simulink model "final_test1"  (Simulink 7.7)
settings: Solver=ode45  StartTime=0.0  StopTime=10.0  RelTol=1e-3
undefined symbols (not defined in the file): des_attributefunction_support, des_figposition
libraries: simeventsattributes2 x107, simeventsserver1 x73, simeventstranslate1 x43, simeventsrouting1 x28, commrandsrc2 x18, simeventsgenerators1 x12, simeventssink1 x9, simeventsqueue1 x6, simulink_extras x1, simeventssignalmanage1 x1
(part 3 of 5)

== system final_test1/Red Link2 ==
  Attribute Function : Subsystem  LoadFcn=des_attributefunction_support(gcb,'LoadFcn');  StartFcn=des_attributefunction_support(gcb,'StartFcn');  mask(Attribute Function){OutputNamePrefix=out_}
      mask prompts: OutputNamePrefix "Prefix name"
      settings: CopyFcn=des_attributefunction_support(gcb,'CopyFcn');  OpenFcn=des_attributefunction_support(gcb,'OpenFcn');  ErrorFcn=des_error_redirect
      mask Help: helpview(simeventsbhelp('attributefunction'))
      mask Display: image(des_iconLoad('attribFunction.jpg'),'center');
  Attribute Function1 : Subsystem  LoadFcn=des_attributefunction_support(gcb,'LoadFcn');  StartFcn=des_attributefunction_support(gcb,'StartFcn');  mask(Attribute Function){OutputNamePrefix=out_}
      mask prompts: OutputNamePrefix "Prefix name"
      settings: CopyFcn=des_attributefunction_support(gcb,'CopyFcn');  OpenFcn=des_attributefunction_support(gcb,'OpenFcn');  ErrorFcn=des_error_redirect
      mask Help: helpview(simeventsbhelp('attributefunction'))
      mask Display: image(des_iconLoad('attribFunction.jpg'),'center');
  Infinite Server : simeventsserver1/Infinite Server  SystemSampleTime=-1  ServiceTimeFrom=Dialog  ServiceTime=0.001  AttributeName=ServiceTime  PriorityServiceCompletion=500  EnableTOPort=off  StatNumberDeparted=Off  StatNumberInBlock=Off  StatPendingEntity=Off  StatNumberPending=Off  StatAverageWait=Off  StatNumberTimedout=Off
  Infinite Server1 : simeventsserver1/Infinite Server  SystemSampleTime=-1  ServiceTimeFrom=Dialog  ServiceTime=0.001  AttributeName=ServiceTime  PriorityServiceCompletion=500  EnableTOPort=off  StatNumberDeparted=Off  StatNumberInBlock=Off  StatPendingEntity=Off  StatNumberPending=Off  StatAverageWait=Off  StatNumberTimedout=Off
  Single Server : simeventsserver1/Single Server  SystemSampleTime=-1  ServiceTimeFrom=Attribute  ServiceTime=1  AttributeName=ServiceTime  PriorityServiceCompletion=500  PermitPreemption=off  SortingAttributeName=PriorityAttributeName  SortingDirection=Ascending  WriteToAttribute=off  ResidualAttributeName=ResidualServiceTime  CreateAttribute=on  EnableTOPort=off  StatNumberDeparted=Off  StatNumberInBlock=Off  StatNumberPreempted=Off  StatPendingEntity=Off  StatAverageWait=Off  StatUtilization=Off  StatNumberTimedout=Off
  Single Server1 : simeventsserver1/Single Server  SystemSampleTime=-1  ServiceTimeFrom=Attribute  ServiceTime=1  AttributeName=ServiceTime  PriorityServiceCompletion=500  PermitPreemption=off  SortingAttributeName=PriorityAttributeName  SortingDirection=Ascending  WriteToAttribute=off  ResidualAttributeName=ResidualServiceTime  CreateAttribute=on  EnableTOPort=off  StatNumberDeparted=Off  StatNumberInBlock=Off  StatNumberPreempted=Off  StatPendingEntity=Off  StatAverageWait=Off  StatUtilization=Off  StatNumberTimedout=Off
  Input1 : PMIOPort  Port=1  Side=Left
  Output1 : PMIOPort  Port=2  Side=Right
  Input2 : PMIOPort  Port=3  Side=Right
  Output2 : PMIOPort  Port=4  Side=Left
  connections:
  Input1/RConn1 -- Attribute Function/LConn1
  Output1/RConn1 -- Infinite Server1/RConn1
  Output2/RConn1 -- Infinite Server/RConn1
  Attribute Function/RConn1 -- Single Server/LConn1
  Single Server/RConn1 -- Infinite Server1/LConn1
  Single Server1/RConn1 -- Infinite Server/LConn1
  Input2/RConn1 -- Attribute Function1/LConn1
  Attribute Function1/RConn1 -- Single Server1/LConn1

== system final_test1/Red Link3 ==
  Attribute Function : Subsystem  LoadFcn=des_attributefunction_support(gcb,'LoadFcn');  StartFcn=des_attributefunction_support(gcb,'StartFcn');  mask(Attribute Function){OutputNamePrefix=out_}
      mask prompts: OutputNamePrefix "Prefix name"
      settings: CopyFcn=des_attributefunction_support(gcb,'CopyFcn');  OpenFcn=des_attributefunction_support(gcb,'OpenFcn');  ErrorFcn=des_error_redirect
      mask Help: helpview(simeventsbhelp('attributefunction'))
      mask Display: image(des_iconLoad('attribFunction.jpg'),'center');
  Attribute Function1 : Subsystem  LoadFcn=des_attributefunction_support(gcb,'LoadFcn');  StartFcn=des_attributefunction_support(gcb,'StartFcn');  mask(Attribute Function){OutputNamePrefix=out_}
      mask prompts: OutputNamePrefix "Prefix name"
      settings: CopyFcn=des_attributefunction_support(gcb,'CopyFcn');  OpenFcn=des_attributefunction_support(gcb,'OpenFcn');  ErrorFcn=des_error_redirect
      mask Help: helpview(simeventsbhelp('attributefunction'))
      mask Display: image(des_iconLoad('attribFunction.jpg'),'center');
  Infinite Server : simeventsserver1/Infinite Server  SystemSampleTime=-1  ServiceTimeFrom=Dialog  ServiceTime=0.001  AttributeName=ServiceTime  PriorityServiceCompletion=500  EnableTOPort=off  StatNumberDeparted=Off  StatNumberInBlock=Off  StatPendingEntity=Off  StatNumberPending=Off  StatAverageWait=Off  StatNumberTimedout=Off
  Infinite Server1 : simeventsserver1/Infinite Server  SystemSampleTime=-1  ServiceTimeFrom=Dialog  ServiceTime=0.001  AttributeName=ServiceTime  PriorityServiceCompletion=500  EnableTOPort=off  StatNumberDeparted=Off  StatNumberInBlock=Off  StatPendingEntity=Off  StatNumberPending=Off  StatAverageWait=Off  StatNumberTimedout=Off
  Single Server : simeventsserver1/Single Server  SystemSampleTime=-1  ServiceTimeFrom=Attribute  ServiceTime=1  AttributeName=ServiceTime  PriorityServiceCompletion=500  PermitPreemption=off  SortingAttributeName=PriorityAttributeName  SortingDirection=Ascending  WriteToAttribute=off  ResidualAttributeName=ResidualServiceTime  CreateAttribute=on  EnableTOPort=off  StatNumberDeparted=Off  StatNumberInBlock=Off  StatNumberPreempted=Off  StatPendingEntity=Off  StatAverageWait=Off  StatUtilization=Off  StatNumberTimedout=Off
  Single Server1 : simeventsserver1/Single Server  SystemSampleTime=-1  ServiceTimeFrom=Attribute  ServiceTime=1  AttributeName=ServiceTime  PriorityServiceCompletion=500  PermitPreemption=off  SortingAttributeName=PriorityAttributeName  SortingDirection=Ascending  WriteToAttribute=off  ResidualAttributeName=ResidualServiceTime  CreateAttribute=on  EnableTOPort=off  StatNumberDeparted=Off  StatNumberInBlock=Off  StatNumberPreempted=Off  StatPendingEntity=Off  StatAverageWait=Off  StatUtilization=Off  StatNumberTimedout=Off
  Input1 : PMIOPort  Port=1  Side=Left
  Output1 : PMIOPort  Port=2  Side=Right
  Input2 : PMIOPort  Port=3  Side=Right
  Output2 : PMIOPort  Port=4  Side=Left
  connections:
  Attribute Function1/RConn1 -- Single Server1/LConn1
  Input2/RConn1 -- Attribute Function1/LConn1
  Single Server1/RConn1 -- Infinite Server/LConn1
  Single Server/RConn1 -- Infinite Server1/LConn1
  Attribute Function/RConn1 -- Single Server/LConn1
  Output2/RConn1 -- Infinite Server/RConn1
  Output1/RConn1 -- Infinite Server1/RConn1
  Input1/RConn1 -- Attribute Function/LConn1

== system final_test1/Red Link4 ==
  Attribute Function : Subsystem  LoadFcn=des_attributefunction_support(gcb,'LoadFcn');  StartFcn=des_attributefunction_support(gcb,'StartFcn');  mask(Attribute Function){OutputNamePrefix=out_}
      mask prompts: OutputNamePrefix "Prefix name"
      settings: CopyFcn=des_attributefunction_support(gcb,'CopyFcn');  OpenFcn=des_attributefunction_support(gcb,'OpenFcn');  ErrorFcn=des_error_redirect
      mask Help: helpview(simeventsbhelp('attributefunction'))
      mask Display: image(des_iconLoad('attribFunction.jpg'),'center');
  Attribute Function1 : Subsystem  LoadFcn=des_attributefunction_support(gcb,'LoadFcn');  StartFcn=des_attributefunction_support(gcb,'StartFcn');  mask(Attribute Function){OutputNamePrefix=out_}
      mask prompts: OutputNamePrefix "Prefix name"
      settings: CopyFcn=des_attributefunction_support(gcb,'CopyFcn');  OpenFcn=des_attributefunction_support(gcb,'OpenFcn');  ErrorFcn=des_error_redirect
      mask Help: helpview(simeventsbhelp('attributefunction'))
      mask Display: image(des_iconLoad('attribFunction.jpg'),'center');
  Infinite Server : simeventsserver1/Infinite Server  SystemSampleTime=-1  ServiceTimeFrom=Dialog  ServiceTime=0.001  AttributeName=ServiceTime  PriorityServiceCompletion=500  EnableTOPort=off  StatNumberDeparted=Off  StatNumberInBlock=Off  StatPendingEntity=Off  StatNumberPending=Off  StatAverageWait=Off  StatNumberTimedout=Off
  Infinite Server1 : simeventsserver1/Infinite Server  SystemSampleTime=-1  ServiceTimeFrom=Dialog  ServiceTime=0.001  AttributeName=ServiceTime  PriorityServiceCompletion=500  EnableTOPort=off  StatNumberDeparted=Off  StatNumberInBlock=Off  StatPendingEntity=Off  StatNumberPending=Off  StatAverageWait=Off  StatNumberTimedout=Off
  Single Server : simeventsserver1/Single Server  SystemSampleTime=-1  ServiceTimeFrom=Attribute  ServiceTime=1  AttributeName=ServiceTime  PriorityServiceCompletion=500  PermitPreemption=off  SortingAttributeName=PriorityAttributeName  SortingDirection=Ascending  WriteToAttribute=off  ResidualAttributeName=ResidualServiceTime  CreateAttribute=on  EnableTOPort=off  StatNumberDeparted=Off  StatNumberInBlock=Off  StatNumberPreempted=Off  StatPendingEntity=Off  StatAverageWait=Off  StatUtilization=Off  StatNumberTimedout=Off
  Single Server1 : simeventsserver1/Single Server  SystemSampleTime=-1  ServiceTimeFrom=Attribute  ServiceTime=1  AttributeName=ServiceTime  PriorityServiceCompletion=500  PermitPreemption=off  SortingAttributeName=PriorityAttributeName  SortingDirection=Ascending  WriteToAttribute=off  ResidualAttributeName=ResidualServiceTime  CreateAttribute=on  EnableTOPort=off  StatNumberDeparted=Off  StatNumberInBlock=Off  StatNumberPreempted=Off  StatPendingEntity=Off  StatAverageWait=Off  StatUtilization=Off  StatNumberTimedout=Off
  Input1 : PMIOPort  Port=1  Side=Left
  Output1 : PMIOPort  Port=2  Side=Right
  Input2 : PMIOPort  Port=3  Side=Right
  Output2 : PMIOPort  Port=4  Side=Left
  connections:
  Input1/RConn1 -- Attribute Function/LConn1
  Output1/RConn1 -- Infinite Server1/RConn1
  Output2/RConn1 -- Infinite Server/RConn1
  Attribute Function/RConn1 -- Single Server/LConn1
  Single Server/RConn1 -- Infinite Server1/LConn1
  Single Server1/RConn1 -- Infinite Server/LConn1
  Input2/RConn1 -- Attribute Function1/LConn1
  Attribute Function1/RConn1 -- Single Server1/LConn1

== system final_test1/Red Link5 ==
  Attribute Function : Subsystem  LoadFcn=des_attributefunction_support(gcb,'LoadFcn');  StartFcn=des_attributefunction_support(gcb,'StartFcn');  mask(Attribute Function){OutputNamePrefix=out_}
      mask prompts: OutputNamePrefix "Prefix name"
      settings: CopyFcn=des_attributefunction_support(gcb,'CopyFcn');  OpenFcn=des_attributefunction_support(gcb,'OpenFcn');  ErrorFcn=des_error_redirect
      mask Help: helpview(simeventsbhelp('attributefunction'))
      mask Display: image(des_iconLoad('attribFunction.jpg'),'center');
  Attribute Function1 : Subsystem  LoadFcn=des_attributefunction_support(gcb,'LoadFcn');  StartFcn=des_attributefunction_support(gcb,'StartFcn');  mask(Attribute Function){OutputNamePrefix=out_}
      mask prompts: OutputNamePrefix "Prefix name"
      settings: CopyFcn=des_attributefunction_support(gcb,'CopyFcn');  OpenFcn=des_attributefunction_support(gcb,'OpenFcn');  ErrorFcn=des_error_redirect
      mask Help: helpview(simeventsbhelp('attributefunction'))
      mask Display: image(des_iconLoad('attribFunction.jpg'),'center');
  Infinite Server : simeventsserver1/Infinite Server  SystemSampleTime=-1  ServiceTimeFrom=Dialog  ServiceTime=0.001  AttributeName=ServiceTime  PriorityServiceCompletion=500  EnableTOPort=off  StatNumberDeparted=Off  StatNumberInBlock=Off  StatPendingEntity=Off  StatNumberPending=Off  StatAverageWait=Off  StatNumberTimedout=Off
  Infinite Server1 : simeventsserver1/Infinite Server  SystemSampleTime=-1  ServiceTimeFrom=Dialog  ServiceTime=0.001  AttributeName=ServiceTime  PriorityServiceCompletion=500  EnableTOPort=off  StatNumberDeparted=Off  StatNumberInBlock=Off  StatPendingEntity=Off  StatNumberPending=Off  StatAverageWait=Off  StatNumberTimedout=Off
  Single Server : simeventsserver1/Single Server  SystemSampleTime=-1  ServiceTimeFrom=Attribute  ServiceTime=1  AttributeName=ServiceTime  PriorityServiceCompletion=500  PermitPreemption=off  SortingAttributeName=PriorityAttributeName  SortingDirection=Ascending  WriteToAttribute=off  ResidualAttributeName=ResidualServiceTime  CreateAttribute=on  EnableTOPort=off  StatNumberDeparted=Off  StatNumberInBlock=Off  StatNumberPreempted=Off  StatPendingEntity=Off  StatAverageWait=Off  StatUtilization=Off  StatNumberTimedout=Off
  Single Server1 : simeventsserver1/Single Server  SystemSampleTime=-1  ServiceTimeFrom=Attribute  ServiceTime=1  AttributeName=ServiceTime  PriorityServiceCompletion=500  PermitPreemption=off  SortingAttributeName=PriorityAttributeName  SortingDirection=Ascending  WriteToAttribute=off  ResidualAttributeName=ResidualServiceTime  CreateAttribute=on  EnableTOPort=off  StatNumberDeparted=Off  StatNumberInBlock=Off  StatNumberPreempted=Off  StatPendingEntity=Off  StatAverageWait=Off  StatUtilization=Off  StatNumberTimedout=Off
  Input1 : PMIOPort  Port=1  Side=Left
  Output1 : PMIOPort  Port=2  Side=Right
  Input2 : PMIOPort  Port=3  Side=Right
  Output2 : PMIOPort  Port=4  Side=Left
  connections:
  Attribute Function1/RConn1 -- Single Server1/LConn1
  Input2/RConn1 -- Attribute Function1/LConn1
  Single Server1/RConn1 -- Infinite Server/LConn1
  Single Server/RConn1 -- Infinite Server1/LConn1
  Attribute Function/RConn1 -- Single Server/LConn1
  Output2/RConn1 -- Infinite Server/RConn1
  Output1/RConn1 -- Infinite Server1/RConn1
  Input1/RConn1 -- Attribute Function/LConn1

== system final_test1/Blue Link/Attribute Function ==
  Embedded MATLAB Function : Stateflow chart  TreatAsAtomicUnit=on
      settings: PropExecContextOutsideSubsystem=on
  __DEML__EDE2FCE__ : simeventstranslate1/Entity Departure Event to Function-Call Event  Priority=1  SystemSampleTime=-1  TimingFunctionCallF1=Before entity departure  EnableE1Port=off  EnableF2Port=off  TimingFunctionCallF2=Before entity departure  EnableE2Port=off  StatNumberDeparted=Off  StatNumberF1Calls=Off  StatNumberF2Calls=Off  IsInsideAFB=on
  __DEML__GA__ : simeventsattributes2/Get Attribute  Priority=1  SystemSampleTime=-1  AttributeName=length  AttributeMissing=Error  AttributeDefaultValue=1  AttributeSendTiming=Before entity departure  AttributeTreatAsVector=1  StatNumberDeparted=Off  EvaluatedDefaultAttributeValue={[]}
  __DEML__SA__ : simeventsattributes2/Set Attribute  Priority=1  SystemSampleTime=-1  AttributeFrom=Signal port  AttributeName=ServiceTime  AttributeTreatAsVector=1  AttributeValue=1  AttributeCreate=on  StatNumberDeparted=Off  EvaluatedAttributeValue={[]}
  IN : PMIOPort  Port=1  Side=Left
  OUT : PMIOPort  Port=2  Side=Right
  wires:
  __DEML__EDE2FCE__/1 -> Embedded MATLAB Function/Trigger
  __DEML__GA__/1 -> Embedded MATLAB Function/1(length)
  Embedded MATLAB Function/1(out_ServiceTime) -> __DEML__SA__/1
  connections:
  __DEML__EDE2FCE__/RConn1 -- __DEML__SA__/LConn1
  __DEML__GA__/RConn1 -- __DEML__EDE2FCE__/LConn1
  IN/RConn1 -- __DEML__GA__/LConn1
  __DEML__SA__/RConn1 -- OUT/RConn1

== system final_test1/Blue Link/Attribute Function1 ==
  Embedded MATLAB Function : Stateflow chart  TreatAsAtomicUnit=on
      settings: PropExecContextOutsideSubsystem=on
  __DEML__EDE2FCE__ : simeventstranslate1/Entity Departure Event to Function-Call Event  Priority=1  SystemSampleTime=-1  TimingFunctionCallF1=Before entity departure  EnableE1Port=off  EnableF2Port=off  TimingFunctionCallF2=Before entity departure  EnableE2Port=off  StatNumberDeparted=Off  StatNumberF1Calls=Off  StatNumberF2Calls=Off  IsInsideAFB=on
  __DEML__GA__ : simeventsattributes2/Get Attribute  Priority=1  SystemSampleTime=-1  AttributeName=length  AttributeMissing=Error  AttributeDefaultValue=1  AttributeSendTiming=Before entity departure  AttributeTreatAsVector=1  StatNumberDeparted=Off  EvaluatedDefaultAttributeValue={[]}
  __DEML__SA__ : simeventsattributes2/Set Attribute  Priority=1  SystemSampleTime=-1  AttributeFrom=Signal port  AttributeName=ServiceTime  AttributeTreatAsVector=1  AttributeValue=1  AttributeCreate=on  StatNumberDeparted=Off  EvaluatedAttributeValue={[]}
  IN : PMIOPort  Port=1  Side=Left
  OUT : PMIOPort  Port=2  Side=Right
  wires:
  __DEML__EDE2FCE__/1 -> Embedded MATLAB Function/Trigger
  __DEML__GA__/1 -> Embedded MATLAB Function/1(length)
  Embedded MATLAB Function/1(out_ServiceTime) -> __DEML__SA__/1
  connections:
  __DEML__SA__/RConn1 -- OUT/RConn1
  IN/RConn1 -- __DEML__GA__/LConn1
  __DEML__GA__/RConn1 -- __DEML__EDE2FCE__/LConn1
  __DEML__EDE2FCE__/RConn1 -- __DEML__SA__/LConn1

== system final_test1/Blue Link1/Attribute Function ==
  Embedded MATLAB Function : Stateflow chart  TreatAsAtomicUnit=on
      settings: PropExecContextOutsideSubsystem=on
  __DEML__EDE2FCE__ : simeventstranslate1/Entity Departure Event to Function-Call Event  Priority=1  SystemSampleTime=-1  TimingFunctionCallF1=Before entity departure  EnableE1Port=off  EnableF2Port=off  TimingFunctionCallF2=Before entity departure  EnableE2Port=off  StatNumberDeparted=Off  StatNumberF1Calls=Off  StatNumberF2Calls=Off  IsInsideAFB=on
  __DEML__GA__ : simeventsattributes2/Get Attribute  Priority=1  SystemSampleTime=-1  AttributeName=length  AttributeMissing=Error  AttributeDefaultValue=1  AttributeSendTiming=Before entity departure  AttributeTreatAsVector=1  StatNumberDeparted=Off  EvaluatedDefaultAttributeValue={[]}
  __DEML__SA__ : simeventsattributes2/Set Attribute  Priority=1  SystemSampleTime=-1  AttributeFrom=Signal port  AttributeName=ServiceTime  AttributeTreatAsVector=1  AttributeValue=1  AttributeCreate=on  StatNumberDeparted=Off  EvaluatedAttributeValue={[]}
  IN : PMIOPort  Port=1  Side=Left
  OUT : PMIOPort  Port=2  Side=Right
  wires:
  __DEML__EDE2FCE__/1 -> Embedded MATLAB Function/Trigger
  __DEML__GA__/1 -> Embedded MATLAB Function/1(length)
  Embedded MATLAB Function/1(out_ServiceTime) -> __DEML__SA__/1
  connections:
  __DEML__SA__/RConn1 -- OUT/RConn1
  IN/RConn1 -- __DEML__GA__/LConn1
  __DEML__GA__/RConn1 -- __DEML__EDE2FCE__/LConn1
  __DEML__EDE2FCE__/RConn1 -- __DEML__SA__/LConn1

== system final_test1/Blue Link1/Attribute Function1 ==
  Embedded MATLAB Function : Stateflow chart  TreatAsAtomicUnit=on
      settings: PropExecContextOutsideSubsystem=on
  __DEML__EDE2FCE__ : simeventstranslate1/Entity Departure Event to Function-Call Event  Priority=1  SystemSampleTime=-1  TimingFunctionCallF1=Before entity departure  EnableE1Port=off  EnableF2Port=off  TimingFunctionCallF2=Before entity departure  EnableE2Port=off  StatNumberDeparted=Off  StatNumberF1Calls=Off  StatNumberF2Calls=Off  IsInsideAFB=on
  __DEML__GA__ : simeventsattributes2/Get Attribute  Priority=1  SystemSampleTime=-1  AttributeName=length  AttributeMissing=Error  AttributeDefaultValue=1  AttributeSendTiming=Before entity departure  AttributeTreatAsVector=1  StatNumberDeparted=Off  EvaluatedDefaultAttributeValue={[]}
  __DEML__SA__ : simeventsattributes2/Set Attribute  Priority=1  SystemSampleTime=-1  AttributeFrom=Signal port  AttributeName=ServiceTime  AttributeTreatAsVector=1  AttributeValue=1  AttributeCreate=on  StatNumberDeparted=Off  EvaluatedAttributeValue={[]}
  IN : PMIOPort  Port=1  Side=Left
  OUT : PMIOPort  Port=2  Side=Right
  wires:
  __DEML__EDE2FCE__/1 -> Embedded MATLAB Function/Trigger
  __DEML__GA__/1 -> Embedded MATLAB Function/1(length)
  Embedded MATLAB Function/1(out_ServiceTime) -> __DEML__SA__/1
  connections:
  __DEML__EDE2FCE__/RConn1 -- __DEML__SA__/LConn1
  __DEML__GA__/RConn1 -- __DEML__EDE2FCE__/LConn1
  IN/RConn1 -- __DEML__GA__/LConn1
  __DEML__SA__/RConn1 -- OUT/RConn1

== system final_test1/Blue Link2/Attribute Function ==
  Embedded MATLAB Function : Stateflow chart  TreatAsAtomicUnit=on
      settings: PropExecContextOutsideSubsystem=on
  __DEML__EDE2FCE__ : simeventstranslate1/Entity Departure Event to Function-Call Event  Priority=1  SystemSampleTime=-1  TimingFunctionCallF1=Before entity departure  EnableE1Port=off  EnableF2Port=off  TimingFunctionCallF2=Before entity departure  EnableE2Port=off  StatNumberDeparted=Off  StatNumberF1Calls=Off  StatNumberF2Calls=Off  IsInsideAFB=on
  __DEML__GA__ : simeventsattributes2/Get Attribute  Priority=1  SystemSampleTime=-1  AttributeName=length  AttributeMissing=Error  AttributeDefaultValue=1  AttributeSendTiming=Before entity departure  AttributeTreatAsVector=1  StatNumberDeparted=Off  EvaluatedDefaultAttributeValue={[]}
  __DEML__SA__ : simeventsattributes2/Set Attribute  Priority=1  SystemSampleTime=-1  AttributeFrom=Signal port  AttributeName=ServiceTime  AttributeTreatAsVector=1  AttributeValue=1  AttributeCreate=on  StatNumberDeparted=Off  EvaluatedAttributeValue={[]}
  IN : PMIOPort  Port=1  Side=Left
  OUT : PMIOPort  Port=2  Side=Right
  wires:
  __DEML__EDE2FCE__/1 -> Embedded MATLAB Function/Trigger
  __DEML__GA__/1 -> Embedded MATLAB Function/1(length)
  Embedded MATLAB Function/1(out_ServiceTime) -> __DEML__SA__/1
  connections:
  __DEML__EDE2FCE__/RConn1 -- __DEML__SA__/LConn1
  __DEML__GA__/RConn1 -- __DEML__EDE2FCE__/LConn1
  IN/RConn1 -- __DEML__GA__/LConn1
  __DEML__SA__/RConn1 -- OUT/RConn1

== system final_test1/Blue Link2/Attribute Function1 ==
  Embedded MATLAB Function : Stateflow chart  TreatAsAtomicUnit=on
      settings: PropExecContextOutsideSubsystem=on
  __DEML__EDE2FCE__ : simeventstranslate1/Entity Departure Event to Function-Call Event  Priority=1  SystemSampleTime=-1  TimingFunctionCallF1=Before entity departure  EnableE1Port=off  EnableF2Port=off  TimingFunctionCallF2=Before entity departure  EnableE2Port=off  StatNumberDeparted=Off  StatNumberF1Calls=Off  StatNumberF2Calls=Off  IsInsideAFB=on
  __DEML__GA__ : simeventsattributes2/Get Attribute  Priority=1  SystemSampleTime=-1  AttributeName=length  AttributeMissing=Error  AttributeDefaultValue=1  AttributeSendTiming=Before entity departure  AttributeTreatAsVector=1  StatNumberDeparted=Off  EvaluatedDefaultAttributeValue={[]}
  __DEML__SA__ : simeventsattributes2/Set Attribute  Priority=1  SystemSampleTime=-1  AttributeFrom=Signal port  AttributeName=ServiceTime  AttributeTreatAsVector=1  AttributeValue=1  AttributeCreate=on  StatNumberDeparted=Off  EvaluatedAttributeValue={[]}
  IN : PMIOPort  Port=1  Side=Left
  OUT : PMIOPort  Port=2  Side=Right
  wires:
  __DEML__EDE2FCE__/1 -> Embedded MATLAB Function/Trigger
  __DEML__GA__/1 -> Embedded MATLAB Function/1(length)
  Embedded MATLAB Function/1(out_ServiceTime) -> __DEML__SA__/1
  connections:
  __DEML__SA__/RConn1 -- OUT/RConn1
  IN/RConn1 -- __DEML__GA__/LConn1
  __DEML__GA__/RConn1 -- __DEML__EDE2FCE__/LConn1
  __DEML__EDE2FCE__/RConn1 -- __DEML__SA__/LConn1

== system final_test1/Blue Link3/Attribute Function ==
  Embedded MATLAB Function : Stateflow chart  TreatAsAtomicUnit=on
      settings: PropExecContextOutsideSubsystem=on
  __DEML__EDE2FCE__ : simeventstranslate1/Entity Departure Event to Function-Call Event  Priority=1  SystemSampleTime=-1  TimingFunctionCallF1=Before entity departure  EnableE1Port=off  EnableF2Port=off  TimingFunctionCallF2=Before entity departure  EnableE2Port=off  StatNumberDeparted=Off  StatNumberF1Calls=Off  StatNumberF2Calls=Off  IsInsideAFB=on
  __DEML__GA__ : simeventsattributes2/Get Attribute  Priority=1  SystemSampleTime=-1  AttributeName=length  AttributeMissing=Error  AttributeDefaultValue=1  AttributeSendTiming=Before entity departure  AttributeTreatAsVector=1  StatNumberDeparted=Off  EvaluatedDefaultAttributeValue={[]}
  __DEML__SA__ : simeventsattributes2/Set Attribute  Priority=1  SystemSampleTime=-1  AttributeFrom=Signal port  AttributeName=ServiceTime  AttributeTreatAsVector=1  AttributeValue=1  AttributeCreate=on  StatNumberDeparted=Off  EvaluatedAttributeValue={[]}
  IN : PMIOPort  Port=1  Side=Left
  OUT : PMIOPort  Port=2  Side=Right
  wires:
  __DEML__EDE2FCE__/1 -> Embedded MATLAB Function/Trigger
  __DEML__GA__/1 -> Embedded MATLAB Function/1(length)
  Embedded MATLAB Function/1(out_ServiceTime) -> __DEML__SA__/1
  connections:
  __DEML__SA__/RConn1 -- OUT/RConn1
  IN/RConn1 -- __DEML__GA__/LConn1
  __DEML__GA__/RConn1 -- __DEML__EDE2FCE__/LConn1
  __DEML__EDE2FCE__/RConn1 -- __DEML__SA__/LConn1

== system final_test1/Blue Link3/Attribute Function1 ==
  Embedded MATLAB Function : Stateflow chart  TreatAsAtomicUnit=on
      settings: PropExecContextOutsideSubsystem=on
  __DEML__EDE2FCE__ : simeventstranslate1/Entity Departure Event to Function-Call Event  Priority=1  SystemSampleTime=-1  TimingFunctionCallF1=Before entity departure  EnableE1Port=off  EnableF2Port=off  TimingFunctionCallF2=Before entity departure  EnableE2Port=off  StatNumberDeparted=Off  StatNumberF1Calls=Off  StatNumberF2Calls=Off  IsInsideAFB=on
  __DEML__GA__ : simeventsattributes2/Get Attribute  Priority=1  SystemSampleTime=-1  AttributeName=length  AttributeMissing=Error  AttributeDefaultValue=1  AttributeSendTiming=Before entity departure  AttributeTreatAsVector=1  StatNumberDeparted=Off  EvaluatedDefaultAttributeValue={[]}
  __DEML__SA__ : simeventsattributes2/Set Attribute  Priority=1  SystemSampleTime=-1  AttributeFrom=Signal port  AttributeName=ServiceTime  AttributeTreatAsVector=1  AttributeValue=1  AttributeCreate=on  StatNumberDeparted=Off  EvaluatedAttributeValue={[]}
  IN : PMIOPort  Port=1  Side=Left
  OUT : PMIOPort  Port=2  Side=Right
  wires:
  __DEML__EDE2FCE__/1 -> Embedded MATLAB Function/Trigger
  __DEML__GA__/1 -> Embedded MATLAB Function/1(length)
  Embedded MATLAB Function/1(out_ServiceTime) -> __DEML__SA__/1
  connections:
  __DEML__EDE2FCE__/RConn1 -- __DEML__SA__/LConn1
  __DEML__GA__/RConn1 -- __DEML__EDE2FCE__/LConn1
  IN/RConn1 -- __DEML__GA__/LConn1
  __DEML__SA__/RConn1 -- OUT/RConn1

== system final_test1/Green Link/Attribute Function ==
  Embedded MATLAB Function : Stateflow chart  TreatAsAtomicUnit=on
      settings: PropExecContextOutsideSubsystem=on
  __DEML__EDE2FCE__ : simeventstranslate1/Entity Departure Event to Function-Call Event  Priority=1  SystemSampleTime=-1  TimingFunctionCallF1=Before entity departure  EnableE1Port=off  EnableF2Port=off  TimingFunctionCallF2=Before entity departure  EnableE2Port=off  StatNumberDeparted=Off  StatNumberF1Calls=Off  StatNumberF2Calls=Off  IsInsideAFB=on
  __DEML__GA__ : simeventsattributes2/Get Attribute  Priority=1  SystemSampleTime=-1  AttributeName=length  AttributeMissing=Error  AttributeDefaultValue=1  AttributeSendTiming=Before entity departure  AttributeTreatAsVector=1  StatNumberDeparted=Off  EvaluatedDefaultAttributeValue={[]}
  __DEML__SA__ : simeventsattributes2/Set Attribute  Priority=1  SystemSampleTime=-1  AttributeFrom=Signal port  AttributeName=ServiceTime  AttributeTreatAsVector=1  AttributeValue=1  AttributeCreate=on  StatNumberDeparted=Off  EvaluatedAttributeValue={[]}
  IN : PMIOPort  Port=1  Side=Left
  OUT : PMIOPort  Port=2  Side=Right
  wires:
  __DEML__EDE2FCE__/1 -> Embedded MATLAB Function/Trigger
  __DEML__GA__/1 -> Embedded MATLAB Function/1(length)
  Embedded MATLAB Function/1(out_ServiceTime) -> __DEML__SA__/1
  connections:
  __DEML__EDE2FCE__/RConn1 -- __DEML__SA__/LConn1
  __DEML__GA__/RConn1 -- __DEML__EDE2FCE__/LConn1
  IN/RConn1 -- __DEML__GA__/LConn1
  __DEML__SA__/RConn1 -- OUT/RConn1

== system final_test1/Green Link/Attribute Function1 ==
  Embedded MATLAB Function : Stateflow chart  TreatAsAtomicUnit=on
      settings: PropExecContextOutsideSubsystem=on
  __DEML__EDE2FCE__ : simeventstranslate1/Entity Departure Event to Function-Call Event  Priority=1  SystemSampleTime=-1  TimingFunctionCallF1=Before entity departure  EnableE1Port=off  EnableF2Port=off  TimingFunctionCallF2=Before entity departure  EnableE2Port=off  StatNumberDeparted=Off  StatNumberF1Calls=Off  StatNumberF2Calls=Off  IsInsideAFB=on
  __DEML__GA__ : simeventsattributes2/Get Attribute  Priority=1  SystemSampleTime=-1  AttributeName=length  AttributeMissing=Error  AttributeDefaultValue=1  AttributeSendTiming=Before entity departure  AttributeTreatAsVector=1  StatNumberDeparted=Off  EvaluatedDefaultAttributeValue={[]}
  __DEML__SA__ : simeventsattributes2/Set Attribute  Priority=1  SystemSampleTime=-1  AttributeFrom=Signal port  AttributeName=ServiceTime  AttributeTreatAsVector=1  AttributeValue=1  AttributeCreate=on  StatNumberDeparted=Off  EvaluatedAttributeValue={[]}
  IN : PMIOPort  Port=1  Side=Left
  OUT : PMIOPort  Port=2  Side=Right
  wires:
  __DEML__EDE2FCE__/1 -> Embedded MATLAB Function/Trigger
  __DEML__GA__/1 -> Embedded MATLAB Function/1(length)
  Embedded MATLAB Function/1(out_ServiceTime) -> __DEML__SA__/1
  connections:
  __DEML__SA__/RConn1 -- OUT/RConn1
  IN/RConn1 -- __DEML__GA__/LConn1
  __DEML__GA__/RConn1 -- __DEML__EDE2FCE__/LConn1
  __DEML__EDE2FCE__/RConn1 -- __DEML__SA__/LConn1

== system final_test1/Green Link1/Attribute Function ==
  Embedded MATLAB Function : Stateflow chart  TreatAsAtomicUnit=on
      settings: PropExecContextOutsideSubsystem=on
  __DEML__EDE2FCE__ : simeventstranslate1/Entity Departure Event to Function-Call Event  Priority=1  SystemSampleTime=-1  TimingFunctionCallF1=Before entity departure  EnableE1Port=off  EnableF2Port=off  TimingFunctionCallF2=Before entity departure  EnableE2Port=off  StatNumberDeparted=Off  StatNumberF1Calls=Off  StatNumberF2Calls=Off  IsInsideAFB=on
  __DEML__GA__ : simeventsattributes2/Get Attribute  Priority=1  SystemSampleTime=-1  AttributeName=length  AttributeMissing=Error  AttributeDefaultValue=1  AttributeSendTiming=Before entity departure  AttributeTreatAsVector=1  StatNumberDeparted=Off  EvaluatedDefaultAttributeValue={[]}
  __DEML__SA__ : simeventsattributes2/Set Attribute  Priority=1  SystemSampleTime=-1  AttributeFrom=Signal port  AttributeName=ServiceTime  AttributeTreatAsVector=1  AttributeValue=1  AttributeCreate=on  StatNumberDeparted=Off  EvaluatedAttributeValue={[]}
  IN : PMIOPort  Port=1  Side=Left
  OUT : PMIOPort  Port=2  Side=Right
  wires:
  Embedded MATLAB Function/1(out_ServiceTime) -> __DEML__SA__/1
  __DEML__GA__/1 -> Embedded MATLAB Function/1(length)
  __DEML__EDE2FCE__/1 -> Embedded MATLAB Function/Trigger
  connections:
  __DEML__SA__/RConn1 -- OUT/RConn1
  IN/RConn1 -- __DEML__GA__/LConn1
  __DEML__GA__/RConn1 -- __DEML__EDE2FCE__/LConn1
  __DEML__EDE2FCE__/RConn1 -- __DEML__SA__/LConn1

== system final_test1/Green Link1/Attribute Function1 ==
  Embedded MATLAB Function : Stateflow chart  TreatAsAtomicUnit=on
      settings: PropExecContextOutsideSubsystem=on
  __DEML__EDE2FCE__ : simeventstranslate1/Entity Departure Event to Function-Call Event  Priority=1  SystemSampleTime=-1  TimingFunctionCallF1=Before entity departure  EnableE1Port=off  EnableF2Port=off  TimingFunctionCallF2=Before entity departure  EnableE2Port=off  StatNumberDeparted=Off  StatNumberF1Calls=Off  StatNumberF2Calls=Off  IsInsideAFB=on
  __DEML__GA__ : simeventsattributes2/Get Attribute  Priority=1  SystemSampleTime=-1  AttributeName=length  AttributeMissing=Error  AttributeDefaultValue=1  AttributeSendTiming=Before entity departure  AttributeTreatAsVector=1  StatNumberDeparted=Off  EvaluatedDefaultAttributeValue={[]}
  __DEML__SA__ : simeventsattributes2/Set Attribute  Priority=1  SystemSampleTime=-1  AttributeFrom=Signal port  AttributeName=ServiceTime  AttributeTreatAsVector=1  AttributeValue=1  AttributeCreate=on  StatNumberDeparted=Off  EvaluatedAttributeValue={[]}
  IN : PMIOPort  Port=1  Side=Left
  OUT : PMIOPort  Port=2  Side=Right
  wires:
  Embedded MATLAB Function/1(out_ServiceTime) -> __DEML__SA__/1
  __DEML__GA__/1 -> Embedded MATLAB Function/1(length)
  __DEML__EDE2FCE__/1 -> Embedded MATLAB Function/Trigger
  connections:
  __DEML__EDE2FCE__/RConn1 -- __DEML__SA__/LConn1
  __DEML__GA__/RConn1 -- __DEML__EDE2FCE__/LConn1
  IN/RConn1 -- __DEML__GA__/LConn1
  __DEML__SA__/RConn1 -- OUT/RConn1

== system final_test1/Green Link2/Attribute Function ==
  Embedded MATLAB Function : Stateflow chart  TreatAsAtomicUnit=on
      settings: PropExecContextOutsideSubsystem=on
  __DEML__EDE2FCE__ : simeventstranslate1/Entity Departure Event to Function-Call Event  Priority=1  SystemSampleTime=-1  TimingFunctionCallF1=Before entity departure  EnableE1Port=off  EnableF2Port=off  TimingFunctionCallF2=Before entity departure  EnableE2Port=off  StatNumberDeparted=Off  StatNumberF1Calls=Off  StatNumberF2Calls=Off  IsInsideAFB=on
  __DEML__GA__ : simeventsattributes2/Get Attribute  Priority=1  SystemSampleTime=-1  AttributeName=length  AttributeMissing=Error  AttributeDefaultValue=1  AttributeSendTiming=Before entity departure  AttributeTreatAsVector=1  StatNumberDeparted=Off  EvaluatedDefaultAttributeValue={[]}
  __DEML__SA__ : simeventsattributes2/Set Attribute  Priority=1  SystemSampleTime=-1  AttributeFrom=Signal port  AttributeName=ServiceTime  AttributeTreatAsVector=1  AttributeValue=1  AttributeCreate=on  StatNumberDeparted=Off  EvaluatedAttributeValue={[]}
  IN : PMIOPort  Port=1  Side=Left
  OUT : PMIOPort  Port=2  Side=Right
  wires:
  __DEML__EDE2FCE__/1 -> Embedded MATLAB Function/Trigger
  __DEML__GA__/1 -> Embedded MATLAB Function/1(length)
  Embedded MATLAB Function/1(out_ServiceTime) -> __DEML__SA__/1
  connections:
  __DEML__EDE2FCE__/RConn1 -- __DEML__SA__/LConn1
  __DEML__GA__/RConn1 -- __DEML__EDE2FCE__/LConn1
  IN/RConn1 -- __DEML__GA__/LConn1
  __DEML__SA__/RConn1 -- OUT/RConn1

== system final_test1/Green Link2/Attribute Function1 ==
  Embedded MATLAB Function : Stateflow chart  TreatAsAtomicUnit=on
      settings: PropExecContextOutsideSubsystem=on
  __DEML__EDE2FCE__ : simeventstranslate1/Entity Departure Event to Function-Call Event  Priority=1  SystemSampleTime=-1  TimingFunctionCallF1=Before entity departure  EnableE1Port=off  EnableF2Port=off  TimingFunctionCallF2=Before entity departure  EnableE2Port=off  StatNumberDeparted=Off  StatNumberF1Calls=Off  StatNumberF2Calls=Off  IsInsideAFB=on
  __DEML__GA__ : simeventsattributes2/Get Attribute  Priority=1  SystemSampleTime=-1  AttributeName=length  AttributeMissing=Error  AttributeDefaultValue=1  AttributeSendTiming=Before entity departure  AttributeTreatAsVector=1  StatNumberDeparted=Off  EvaluatedDefaultAttributeValue={[]}
  __DEML__SA__ : simeventsattributes2/Set Attribute  Priority=1  SystemSampleTime=-1  AttributeFrom=Signal port  AttributeName=ServiceTime  AttributeTreatAsVector=1  AttributeValue=1  AttributeCreate=on  StatNumberDeparted=Off  EvaluatedAttributeValue={[]}
  IN : PMIOPort  Port=1  Side=Left
  OUT : PMIOPort  Port=2  Side=Right
  wires:
  __DEML__EDE2FCE__/1 -> Embedded MATLAB Function/Trigger
  __DEML__GA__/1 -> Embedded MATLAB Function/1(length)
  Embedded MATLAB Function/1(out_ServiceTime) -> __DEML__SA__/1
  connections:
  __DEML__SA__/RConn1 -- OUT/RConn1
  IN/RConn1 -- __DEML__GA__/LConn1
  __DEML__GA__/RConn1 -- __DEML__EDE2FCE__/LConn1
  __DEML__EDE2FCE__/RConn1 -- __DEML__SA__/LConn1

== system final_test1/Green Link3/Attribute Function ==
  Embedded MATLAB Function : Stateflow chart  TreatAsAtomicUnit=on
      settings: PropExecContextOutsideSubsystem=on
  __DEML__EDE2FCE__ : simeventstranslate1/Entity Departure Event to Function-Call Event  Priority=1  SystemSampleTime=-1  TimingFunctionCallF1=Before entity departure  EnableE1Port=off  EnableF2Port=off  TimingFunctionCallF2=Before entity departure  EnableE2Port=off  StatNumberDeparted=Off  StatNumberF1Calls=Off  StatNumberF2Calls=Off  IsInsideAFB=on
  __DEML__GA__ : simeventsattributes2/Get Attribute  Priority=1  SystemSampleTime=-1  AttributeName=length  AttributeMissing=Error  AttributeDefaultValue=1  AttributeSendTiming=Before entity departure  AttributeTreatAsVector=1  StatNumberDeparted=Off  EvaluatedDefaultAttributeValue={[]}
  __DEML__SA__ : simeventsattributes2/Set Attribute  Priority=1  SystemSampleTime=-1  AttributeFrom=Signal port  AttributeName=ServiceTime  AttributeTreatAsVector=1  AttributeValue=1  AttributeCreate=on  StatNumberDeparted=Off  EvaluatedAttributeValue={[]}
  IN : PMIOPort  Port=1  Side=Left
  OUT : PMIOPort  Port=2  Side=Right
  wires:
  __DEML__EDE2FCE__/1 -> Embedded MATLAB Function/Trigger
  __DEML__GA__/1 -> Embedded MATLAB Function/1(length)
  Embedded MATLAB Function/1(out_ServiceTime) -> __DEML__SA__/1
  connections:
  __DEML__EDE2FCE__/RConn1 -- __DEML__SA__/LConn1
  __DEML__GA__/RConn1 -- __DEML__EDE2FCE__/LConn1
  IN/RConn1 -- __DEML__GA__/LConn1
  __DEML__SA__/RConn1 -- OUT/RConn1

== system final_test1/Green Link3/Attribute Function1 ==
  Embedded MATLAB Function : Stateflow chart  TreatAsAtomicUnit=on
      settings: PropExecContextOutsideSubsystem=on
  __DEML__EDE2FCE__ : simeventstranslate1/Entity Departure Event to Function-Call Event  Priority=1  SystemSampleTime=-1  TimingFunctionCallF1=Before entity departure  EnableE1Port=off  EnableF2Port=off  TimingFunctionCallF2=Before entity departure  EnableE2Port=off  StatNumberDeparted=Off  StatNumberF1Calls=Off  StatNumberF2Calls=Off  IsInsideAFB=on
  __DEML__GA__ : simeventsattributes2/Get Attribute  Priority=1  SystemSampleTime=-1  AttributeName=length  AttributeMissing=Error  AttributeDefaultValue=1  AttributeSendTiming=Before entity departure  AttributeTreatAsVector=1  StatNumberDeparted=Off  EvaluatedDefaultAttributeValue={[]}
  __DEML__SA__ : simeventsattributes2/Set Attribute  Priority=1  SystemSampleTime=-1  AttributeFrom=Signal port  AttributeName=ServiceTime  AttributeTreatAsVector=1  AttributeValue=1  AttributeCreate=on  StatNumberDeparted=Off  EvaluatedAttributeValue={[]}
  IN : PMIOPort  Port=1  Side=Left
  OUT : PMIOPort  Port=2  Side=Right
  wires:
  __DEML__EDE2FCE__/1 -> Embedded MATLAB Function/Trigger
  __DEML__GA__/1 -> Embedded MATLAB Function/1(length)
  Embedded MATLAB Function/1(out_ServiceTime) -> __DEML__SA__/1
  connections:
  __DEML__SA__/RConn1 -- OUT/RConn1
  IN/RConn1 -- __DEML__GA__/LConn1
  __DEML__GA__/RConn1 -- __DEML__EDE2FCE__/LConn1
  __DEML__EDE2FCE__/RConn1 -- __DEML__SA__/LConn1

== system final_test1/Green Link4/Attribute Function ==
  Embedded MATLAB Function : Stateflow chart  TreatAsAtomicUnit=on
      settings: PropExecContextOutsideSubsystem=on
  __DEML__EDE2FCE__ : simeventstranslate1/Entity Departure Event to Function-Call Event  Priority=1  SystemSampleTime=-1  TimingFunctionCallF1=Before entity departure  EnableE1Port=off  EnableF2Port=off  TimingFunctionCallF2=Before entity departure  EnableE2Port=off  StatNumberDeparted=Off  StatNumberF1Calls=Off  StatNumberF2Calls=Off  IsInsideAFB=on
  __DEML__GA__ : simeventsattributes2/Get Attribute  Priority=1  SystemSampleTime=-1  AttributeName=length  AttributeMissing=Error  AttributeDefaultValue=1  AttributeSendTiming=Before entity departure  AttributeTreatAsVector=1  StatNumberDeparted=Off  EvaluatedDefaultAttributeValue={[]}
  __DEML__SA__ : simeventsattributes2/Set Attribute  Priority=1  SystemSampleTime=-1  AttributeFrom=Signal port  AttributeName=ServiceTime  AttributeTreatAsVector=1  AttributeValue=1  AttributeCreate=on  StatNumberDeparted=Off  EvaluatedAttributeValue={[]}
  IN : PMIOPort  Port=1  Side=Left
  OUT : PMIOPort  Port=2  Side=Right
  wires:
  Embedded MATLAB Function/1(out_ServiceTime) -> __DEML__SA__/1
  __DEML__GA__/1 -> Embedded MATLAB Function/1(length)
  __DEML__EDE2FCE__/1 -> Embedded MATLAB Function/Trigger
  connections:
  __DEML__SA__/RConn1 -- OUT/RConn1
  IN/RConn1 -- __DEML__GA__/LConn1
  __DEML__GA__/RConn1 -- __DEML__EDE2FCE__/LConn1
  __DEML__EDE2FCE__/RConn1 -- __DEML__SA__/LConn1

== system final_test1/Green Link4/Attribute Function1 ==
  Embedded MATLAB Function : Stateflow chart  TreatAsAtomicUnit=on
      settings: PropExecContextOutsideSubsystem=on
  __DEML__EDE2FCE__ : simeventstranslate1/Entity Departure Event to Function-Call Event  Priority=1  SystemSampleTime=-1  TimingFunctionCallF1=Before entity departure  EnableE1Port=off  EnableF2Port=off  TimingFunctionCallF2=Before entity departure  EnableE2Port=off  StatNumberDeparted=Off  StatNumberF1Calls=Off  StatNumberF2Calls=Off  IsInsideAFB=on
  __DEML__GA__ : simeventsattributes2/Get Attribute  Priority=1  SystemSampleTime=-1  AttributeName=length  AttributeMissing=Error  AttributeDefaultValue=1  AttributeSendTiming=Before entity departure  AttributeTreatAsVector=1  StatNumberDeparted=Off  EvaluatedDefaultAttributeValue={[]}
  __DEML__SA__ : simeventsattributes2/Set Attribute  Priority=1  SystemSampleTime=-1  AttributeFrom=Signal port  AttributeName=ServiceTime  AttributeTreatAsVector=1  AttributeValue=1  AttributeCreate=on  StatNumberDeparted=Off  EvaluatedAttributeValue={[]}
  IN : PMIOPort  Port=1  Side=Left
  OUT : PMIOPort  Port=2  Side=Right
  wires:
  Embedded MATLAB Function/1(out_ServiceTime) -> __DEML__SA__/1
  __DEML__GA__/1 -> Embedded MATLAB Function/1(length)
  __DEML__EDE2FCE__/1 -> Embedded MATLAB Function/Trigger
  connections:
  __DEML__EDE2FCE__/RConn1 -- __DEML__SA__/LConn1
  __DEML__GA__/RConn1 -- __DEML__EDE2FCE__/LConn1
  IN/RConn1 -- __DEML__GA__/LConn1
  __DEML__SA__/RConn1 -- OUT/RConn1

== system final_test1/Host 1/Attribute Function ==
  Embedded MATLAB Function : Stateflow chart  TreatAsAtomicUnit=on
      settings: PropExecContextOutsideSubsystem=on
  __DEML__EDE2FCE__ : simeventstranslate1/Entity Departure Event to Function-Call Event  Priority=1  SystemSampleTime=-1  TimingFunctionCallF1=Before entity departure  EnableE1Port=off  EnableF2Port=off  TimingFunctionCallF2=Before entity departure  EnableE2Port=off  StatNumberDeparted=Off  StatNumberF1Calls=Off  StatNumberF2Calls=Off  IsInsideAFB=on
  __DEML__GA__ : simeventsattributes2/Get Attribute  Priority=1  SystemSampleTime=-1  AttributeName=type|size  AttributeMissing=Error|Error  AttributeDefaultValue=1|1  AttributeSendTiming=Before entity departure|Before entity departure  AttributeTreatAsVector=1|1  StatNumberDeparted=Off  EvaluatedDefaultAttributeValue={[];[]}
  __DEML__SA__ : simeventsattributes2/Set Attribute  Priority=1  SystemSampleTime=-1  AttributeFrom=Signal port  AttributeName=length  AttributeTreatAsVector=1  AttributeValue=1  AttributeCreate=on  StatNumberDeparted=Off  EvaluatedAttributeValue={[]}
  IN : PMIOPort  Port=1  Side=Left
  OUT : PMIOPort  Port=2  Side=Right
  wires:
  __DEML__EDE2FCE__/1 -> Embedded MATLAB Function/Trigger
  __DEML__GA__/1 -> Embedded MATLAB Function/1(type)
  __DEML__GA__/2 -> Embedded MATLAB Function/2(size)
  Embedded MATLAB Function/1(out_length) -> __DEML__SA__/1
  connections:
  __DEML__SA__/RConn1 -- OUT/RConn1
  IN/RConn1 -- __DEML__GA__/LConn1
  __DEML__GA__/RConn1 -- __DEML__EDE2FCE__/LConn1
  __DEML__EDE2FCE__/RConn1 -- __DEML__SA__/LConn1

== system final_test1/Host 2/Attribute Function ==
  Embedded MATLAB Function : Stateflow chart  TreatAsAtomicUnit=on
      settings: PropExecContextOutsideSubsystem=on
  __DEML__EDE2FCE__ : simeventstranslate1/Entity Departure Event to Function-Call Event  Priority=1  SystemSampleTime=-1  TimingFunctionCallF1=Before entity departure  EnableE1Port=off  EnableF2Port=off  TimingFunctionCallF2=Before entity departure  EnableE2Port=off  StatNumberDeparted=Off  StatNumberF1Calls=Off  StatNumberF2Calls=Off  IsInsideAFB=on
  __DEML__GA__ : simeventsattributes2/Get Attribute  Priority=1  SystemSampleTime=-1  AttributeName=type|size  AttributeMissing=Error|Error  AttributeDefaultValue=1|1  AttributeSendTiming=Before entity departure|Before entity departure  AttributeTreatAsVector=1|1  StatNumberDeparted=Off  EvaluatedDefaultAttributeValue={[];[]}
  __DEML__SA__ : simeventsattributes2/Set Attribute  Priority=1  SystemSampleTime=-1  AttributeFrom=Signal port  AttributeName=length  AttributeTreatAsVector=1  AttributeValue=1  AttributeCreate=on  StatNumberDeparted=Off  EvaluatedAttributeValue={[]}
  IN : PMIOPort  Port=1  Side=Left
  OUT : PMIOPort  Port=2  Side=Right
  wires:
  __DEML__EDE2FCE__/1 -> Embedded MATLAB Function/Trigger
  __DEML__GA__/1 -> Embedded MATLAB Function/1(type)
  __DEML__GA__/2 -> Embedded MATLAB Function/2(size)
  Embedded MATLAB Function/1(out_length) -> __DEML__SA__/1
  connections:
  __DEML__EDE2FCE__/RConn1 -- __DEML__SA__/LConn1
  __DEML__GA__/RConn1 -- __DEML__EDE2FCE__/LConn1
  IN/RConn1 -- __DEML__GA__/LConn1
  __DEML__SA__/RConn1 -- OUT/RConn1

== system final_test1/Host 3/Attribute Function ==
  Embedded MATLAB Function : Stateflow chart  TreatAsAtomicUnit=on
      settings: PropExecContextOutsideSubsystem=on
  __DEML__EDE2FCE__ : simeventstranslate1/Entity Departure Event to Function-Call Event  Priority=1  SystemSampleTime=-1  TimingFunctionCallF1=Before entity departure  EnableE1Port=off  EnableF2Port=off  TimingFunctionCallF2=Before entity departure  EnableE2Port=off  StatNumberDeparted=Off  StatNumberF1Calls=Off  StatNumberF2Calls=Off  IsInsideAFB=on
  __DEML__GA__ : simeventsattributes2/Get Attribute  Priority=1  SystemSampleTime=-1  AttributeName=type|size  AttributeMissing=Error|Error  AttributeDefaultValue=1|1  AttributeSendTiming=Before entity departure|Before entity departure  AttributeTreatAsVector=1|1  StatNumberDeparted=Off  EvaluatedDefaultAttributeValue={[];[]}
  __DEML__SA__ : simeventsattributes2/Set Attribute  Priority=1  SystemSampleTime=-1  AttributeFrom=Signal port  AttributeName=length  AttributeTreatAsVector=1  AttributeValue=1  AttributeCreate=on  StatNumberDeparted=Off  EvaluatedAttributeValue={[]}
  IN : PMIOPort  Port=1  Side=Left
  OUT : PMIOPort  Port=2  Side=Right
  wires:
  __DEML__EDE2FCE__/1 -> Embedded MATLAB Function/Trigger
  __DEML__GA__/1 -> Embedded MATLAB Function/1(type)
  __DEML__GA__/2 -> Embedded MATLAB Function/2(size)
  Embedded MATLAB Function/1(out_length) -> __DEML__SA__/1
  connections:
  __DEML__SA__/RConn1 -- OUT/RConn1
  IN/RConn1 -- __DEML__GA__/LConn1
  __DEML__GA__/RConn1 -- __DEML__EDE2FCE__/LConn1
  __DEML__EDE2FCE__/RConn1 -- __DEML__SA__/LConn1

== system final_test1/Host 4/Attribute Function ==
  Embedded MATLAB Function : Stateflow chart  TreatAsAtomicUnit=on
      settings: PropExecContextOutsideSubsystem=on
  __DEML__EDE2FCE__ : simeventstranslate1/Entity Departure Event to Function-Call Event  Priority=1  SystemSampleTime=-1  TimingFunctionCallF1=Before entity departure  EnableE1Port=off  EnableF2Port=off  TimingFunctionCallF2=Before entity departure  EnableE2Port=off  StatNumberDeparted=Off  StatNumberF1Calls=Off  StatNumberF2Calls=Off  IsInsideAFB=on
  __DEML__GA__ : simeventsattributes2/Get Attribute  Priority=1  SystemSampleTime=-1  AttributeName=type|size  AttributeMissing=Error|Error  AttributeDefaultValue=1|1  AttributeSendTiming=Before entity departure|Before entity departure  AttributeTreatAsVector=1|1  StatNumberDeparted=Off  EvaluatedDefaultAttributeValue={[];[]}
  __DEML__SA__ : simeventsattributes2/Set Attribute  Priority=1  SystemSampleTime=-1  AttributeFrom=Signal port  AttributeName=length  AttributeTreatAsVector=1  AttributeValue=1  AttributeCreate=on  StatNumberDeparted=Off  EvaluatedAttributeValue={[]}
  IN : PMIOPort  Port=1  Side=Left
  OUT : PMIOPort  Port=2  Side=Right
  wires:
  __DEML__EDE2FCE__/1 -> Embedded MATLAB Function/Trigger
  __DEML__GA__/1 -> Embedded MATLAB Function/1(type)
  __DEML__GA__/2 -> Embedded MATLAB Function/2(size)
  Embedded MATLAB Function/1(out_length) -> __DEML__SA__/1
  connections:
  __DEML__EDE2FCE__/RConn1 -- __DEML__SA__/LConn1
  __DEML__GA__/RConn1 -- __DEML__EDE2FCE__/LConn1
  IN/RConn1 -- __DEML__GA__/LConn1
  __DEML__SA__/RConn1 -- OUT/RConn1

== system final_test1/Host 5/Attribute Function ==
  Embedded MATLAB Function : Stateflow chart  TreatAsAtomicUnit=on
      settings: PropExecContextOutsideSubsystem=on
  __DEML__EDE2FCE__ : simeventstranslate1/Entity Departure Event to Function-Call Event  Priority=1  SystemSampleTime=-1  TimingFunctionCallF1=Before entity departure  EnableE1Port=off  EnableF2Port=off  TimingFunctionCallF2=Before entity departure  EnableE2Port=off  StatNumberDeparted=Off  StatNumberF1Calls=Off  StatNumberF2Calls=Off  IsInsideAFB=on
  __DEML__GA__ : simeventsattributes2/Get Attribute  Priority=1  SystemSampleTime=-1  AttributeName=type|size  AttributeMissing=Error|Error  AttributeDefaultValue=1|1  AttributeSendTiming=Before entity departure|Before entity departure  AttributeTreatAsVector=1|1  StatNumberDeparted=Off  EvaluatedDefaultAttributeValue={[];[]}
  __DEML__SA__ : simeventsattributes2/Set Attribute  Priority=1  SystemSampleTime=-1  AttributeFrom=Signal port  AttributeName=length  AttributeTreatAsVector=1  AttributeValue=1  AttributeCreate=on  StatNumberDeparted=Off  EvaluatedAttributeValue={[]}
  IN : PMIOPort  Port=1  Side=Left
  OUT : PMIOPort  Port=2  Side=Right
  wires:
  __DEML__EDE2FCE__/1 -> Embedded MATLAB Function/Trigger
  __DEML__GA__/1 -> Embedded MATLAB Function/1(type)
  __DEML__GA__/2 -> Embedded MATLAB Function/2(size)
  Embedded MATLAB Function/1(out_length) -> __DEML__SA__/1
  connections:
  __DEML__SA__/RConn1 -- OUT/RConn1
  IN/RConn1 -- __DEML__GA__/LConn1
  __DEML__GA__/RConn1 -- __DEML__EDE2FCE__/LConn1
  __DEML__EDE2FCE__/RConn1 -- __DEML__SA__/LConn1
